simulink model "4_Fullycontrolled_rectifier"  (R2014a)
settings: Solver=ode23tb  StartTime=0.0  StopTime=0.06  RelTol=1e-6
libraries: powerlib x13, powerlib_meascontrol x1
settings Model: Creator=CHANDRA BABU  LastModifiedBy=Divya M
settings SolverCC: ZeroCrossControl=DisableAll
settings DataIOCC: SignalLoggingSaveFormat=ModelDataLogs
settings OptimizationCC: ExpressionDepthLimit=2147483647
settings DebuggingCC: UnderspecifiedInitializationDetection=Classic  FcnCallInpInsideContextMsg=UseLocalSettings  StateNameClashWarn=warning
settings GRTTargetCC: CombineOutputUpdateFcns=off  GRTInterface=on

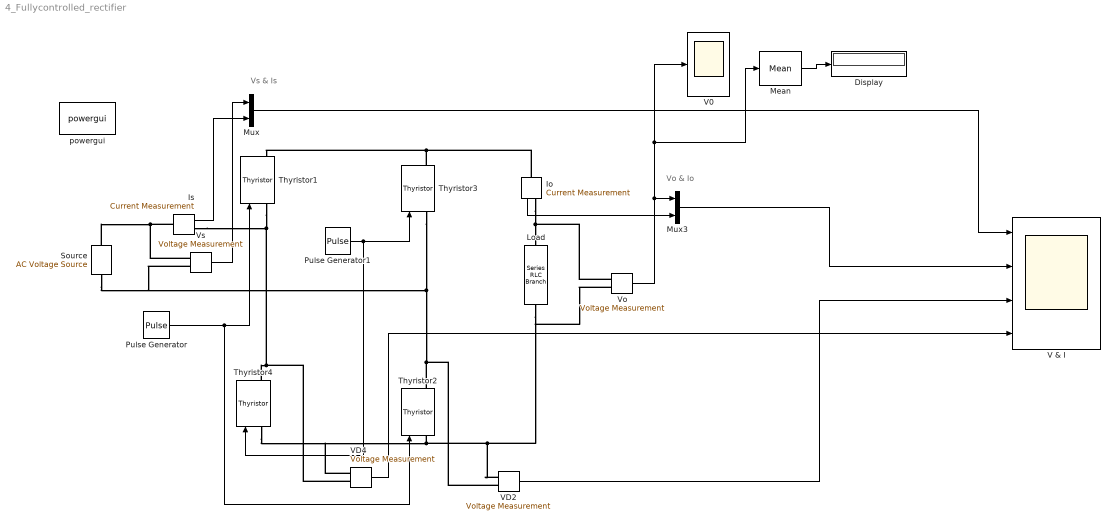
== system 4_Fullycontrolled_rectifier ==
  note: Vo & Io
  note: Vs & Is
  " Source" : powerlib/Electrical Sources/AC Voltage Source  Amplitude=5  Phase=0  Frequency=50  SampleTime=0  Measurements=None
  Display : Display
  Io : powerlib/Measurements/Current Measurement  PhasorSimulation=off  OutputType=Complex  PSBequivalent=0
  Is : powerlib/Measurements/Current Measurement  PhasorSimulation=off  OutputType=Complex  PSBequivalent=0
  Load : powerlib/Elements/Series RLC Branch  LConnTagsString=__new0  RConnTagsString=__new0  BranchType=R  Resistance=2.5  Inductance=1e-3  SetiL0=off  InitialCurrent=0  Capacitance=1e-6  Setx0=off  InitialVoltage=0  Measurements=None
  Mean : powerlib_meascontrol/Measurements/Mean  Freq=60  Vinit=0  Ts=0
  Mux : Mux  Inputs=2
  Mux3 : Mux  Inputs=2
  Pulse Generator : DiscretePulseGenerator  PulseType=Time based  Period=0.02  PulseWidth=5  PhaseDelay=0.005
  Pulse Generator1 : DiscretePulseGenerator  PulseType=Time based  Period=0.02  PulseWidth=5  PhaseDelay=0.015
  Thyristor{1..4} (4 alike) : powerlib/Power Electronics/Thyristor  Ron=0.001  Lon=0  Vf=0.8  IC=0  Rs=500  Cs=250e-9  Measurements=on
  V & I : Scope  NumInputPorts=4
      settings: YMin=-5~0~-5~-5  YMax=5~5~2~2
  V0 : Scope
      settings: SaveName=Outputvoltage
  VD2 : powerlib/Measurements/Voltage Measurement  PhasorSimulation=off  OutputType=Complex  PSBequivalent=0
  VD4 : powerlib/Measurements/Voltage Measurement  PhasorSimulation=off  OutputType=Complex  PSBequivalent=0
  Vo : powerlib/Measurements/Voltage Measurement  PhasorSimulation=off  OutputType=Complex  PSBequivalent=0
  Vs : powerlib/Measurements/Voltage Measurement  PhasorSimulation=off  OutputType=Complex  PSBequivalent=0
  powergui : powerlib/powergui  Priority=1  SimulationMode=Continuous  SolverType=Tustin  SampleTime=50e-6  frequency=60  SPID=off  DisableSnubberDevices=off  DisableRonSwitches=off  DisableVfSwitches=off  SwTol=0  Interpol=off  DisplayEquations=off  Ts=0  methode=off  frequencyindice=0  Pbase=100e6  ErrMax=1e-4  Iterations=50  UnitsV=kV  UnitsW=MW  FunctionMessages=off  echomessages=off  HookPort=off  EnableUseOfTLC=off  x0status=blocks  RestoreLinks=warning  ResistiveCurrentMeasurement=off  Frange=[0:2:500]  Ylog=off  Xlog=on  ShowGrid=off  save=off  variable=ZData  structure=Outputvoltage  ZoomFFT=on  StartTime=0.0  cycles=1  DisplayStyle=1  fundamental=50  FreqAxis=on  MaxFrequency=1000  frequencyindicesteady=1  RmsSteady=1  display=off
  wires:
  Vo/1 -> Mean/1, V0/1, Mux3/1
  Is/1 -> Mux/2
  Io/1 -> Mux3/2
  Vs/1 -> Mux/1
  Mux/1 -> V & I/1
  Mux3/1 -> V & I/2
  VD2/1 -> V & I/3
  VD4/1 -> V & I/4
  Mean/1 -> Display/1
  Pulse Generator/1 -> Thyristor1/1, Thyristor2/1
  Pulse Generator1/1 -> Thyristor3/1, Thyristor4/1
  connections:
  VD4/LConn2 -- Thyristor4/RConn1 -- Thyristor1/LConn1 -- Is/RConn1
  " Source"/LConn1 -- Vs/LConn2 -- Thyristor3/LConn1 -- Thyristor2/RConn1 -- VD2/LConn2
  Vs/LConn1 -- " Source"/RConn1 -- Is/LConn1
  Vo/LConn1 -- Io/RConn1 -- Load/LConn1
  VD2/LConn1 -- Vo/LConn2 -- Load/RConn1 -- Thyristor2/LConn1 -- Thyristor4/LConn1 -- VD4/LConn1
  Io/LConn1 -- Thyristor3/RConn1 -- Thyristor1/RConn1
